simulink model "controlBlockDevelopment_generic"  (Simulink 8.6)
settings: Solver=ode45  StartTime=0.0  StopTime=60  RelTol=1e-3
undefined symbols (not defined in the file): BMTestRig_continuous_output_fixed_coulomb_asym
libraries: simulink x1, SEA_library_models x1
settings Model: Creator=joern  LastModifiedBy=wesley
settings DataIOCC: SignalLoggingSaveFormat=Dataset
settings OptimizationCC: ExpressionDepthLimit=128
settings DebuggingCC: UnderspecifiedInitializationDetection=Simplified  MergeDetectMultiDrivingBlocksExec=error  FcnCallInpInsideContextMsg=EnableAllAsError  StateNameClashWarn=none
settings GRTTargetCC: CombineOutputUpdateFcns=on  GRTInterface=off

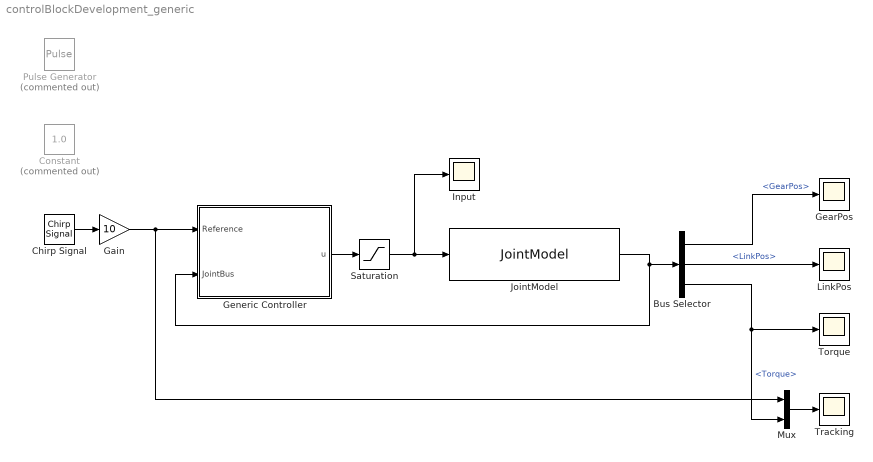
== system controlBlockDevelopment_generic ==
  Bus Selector : BusSelector  OutputSignals=GearPos,LinkPos,Torque
  Chirp Signal : simulink/Sources/Chirp Signal  f1=0.1  T=60  f2=60
  Constant : Constant  Commented=on  Value=1.0
  Gain : Gain  Gain=10
  GearPos : Scope
  Generic Controller : Subsystem  mask{jointObj=BMTestRig_continuous_output_fixed_coulomb_asym}
      mask prompts: jointObj "Joint Object"
      mask init:
      | % Get linear dynamics matrices
      | [A, B, C, I, D, K] = jointObj.getDynamicsMatrices();
  Input : Scope
  JointModel : SEA_library_models/Joint models/JointModel  jointObj=BMTestRig_continuous_output_fixed  fc_vel=100  fc_torque=100  input_delay=0  output_delay=0  input_noise_enabled=off  output_noise_enabled=off  var_u=0.12^2  var_y=1.8e-10
  LinkPos : Scope
  Mux : Mux  Inputs=2
  Pulse Generator : DiscretePulseGenerator  Commented=on  PulseType=Time based  Period=10  PulseWidth=0.1
  Saturation : Saturate  UpperLimit=40  LowerLimit=-40
  Torque : Scope
  Tracking : Scope
  wires:
  JointModel/1 -> Bus Selector/1, Generic Controller/2(JointBus)
  Bus Selector/2 -> LinkPos/1  "<LinkPos>"
  Bus Selector/3 -> Torque/1, Mux/2  "<Torque>"
  Mux/1 -> Tracking/1
  Bus Selector/1 -> GearPos/1  "<GearPos>"
  Chirp Signal/1 -> Gain/1
  Gain/1 -> Generic Controller/1(Reference), Mux/1
  Generic Controller/1(u) -> Saturation/1
  Saturation/1 -> JointModel/1, Input/1

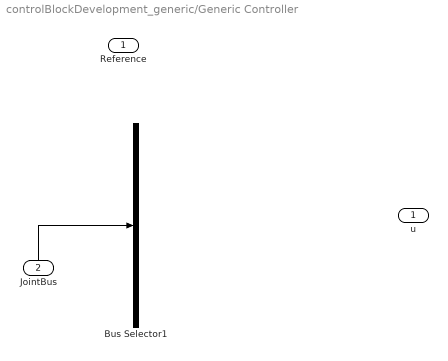
== system controlBlockDevelopment_generic/Generic Controller ==
  Reference : Inport
  JointBus : Inport  Port=2
  Bus Selector1 : BusSelector  OutputSignals=GearPos,LinkPos,Torque
  u : Outport
  wires:
  JointBus/1 -> Bus Selector1/1
